simulink model "untitled2"  (R2018a)
settings: Solver=VariableStepAuto  StartTime=0.0  StopTime=10.0  RelTol=1e-3
undefined symbols (not defined in the file or in its folder): a, b, c, u0, x0
settings Model: Creator=adiravishankara  LastModifiedBy=adiravishankara

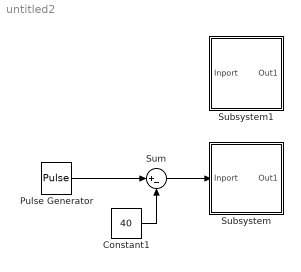
== system untitled2 ==
  Constant1 : Constant  Value=40
  Pulse Generator : DiscretePulseGenerator  PulseType=Time based  Period=10  PulseWidth=5
  Subsystem : Subsystem
  Subsystem1 : Subsystem
  Sum : Sum  Inputs=|+-
  wires:
  Pulse Generator/1 -> Sum/1
  Constant1/1 -> Sum/2
  Sum/1 -> Subsystem/1(Inport)

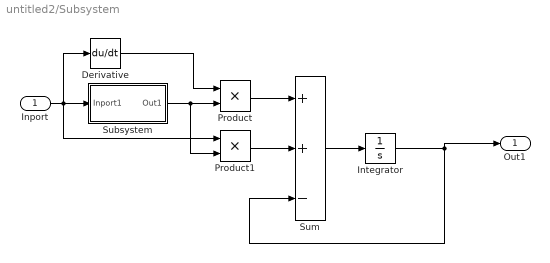
== system untitled2/Subsystem ==
  Inport : Inport
  Derivative : Derivative
  Integrator : Integrator
  Product : Product
  Product1 : Product
  Subsystem : Subsystem
  Sum : Sum  Inputs=++-
  Out1 : Outport
  wires:
  Product/1 -> Sum/1
  Sum/1 -> Integrator/1
  Subsystem/1(Out1) -> Product1/2, Product/2
  Integrator/1 -> Out1/1, Sum/3
  Inport/1 -> Product1/1, Derivative/1, Subsystem/1(Inport1)
  Product1/1 -> Sum/2
  Derivative/1 -> Product/1

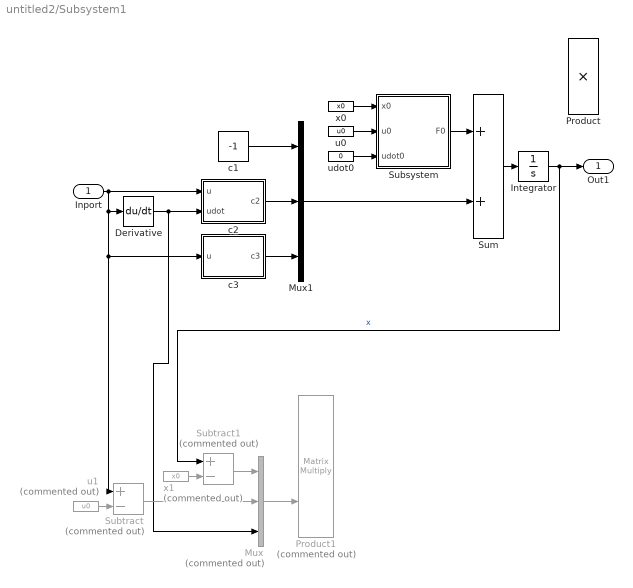
== system untitled2/Subsystem1 ==
  Inport : Inport
  Derivative : Derivative
  Integrator : Integrator
  Mux : Mux  Commented=on  Inputs=3
  Mux1 : Mux  Inputs=3
  Product : Product
  Product1 : Product  Commented=on  Multiplication=Matrix(*)
  Subsystem : Subsystem
  Subtract : Sum  Commented=on  Inputs=+-
  Subtract1 : Sum  Commented=on  Inputs=+-
  Sum : Sum
  c1 : Constant  Value=-1
  c2 : Subsystem
  c3 : Subsystem
  u0 : Constant  Value=u0
  u1 : Constant  Commented=on  Value=u0
  udot0 : Constant  Value=0
  x0 : Constant  Value=x0
  x1 : Constant  Commented=on  Value=x0
  Out1 : Outport
  wires:
  Integrator/1 -> Subtract1/1, Out1/1  "x"
  Sum/1 -> Integrator/1
  Mux/1 -> Product1/2
  Mux1/1 -> Sum/2
  c3/1(c3) -> Mux1/3
  c2/1(c2) -> Mux1/2
  c1/1 -> Mux1/1
  Subsystem/1(F0) -> Sum/1
  udot0/1 -> Subsystem/3(udot0)
  u0/1 -> Subsystem/2(u0)
  x0/1 -> Subsystem/1(x0)
  Inport/1 -> c2/1(u), Subtract/1, c3/1(u), Derivative/1
  Derivative/1 -> Mux/3, c2/2(udot)
  u1/1 -> Subtract/2
  Subtract/1 -> Mux/2
  Subtract1/1 -> Mux/1
  x1/1 -> Subtract1/2

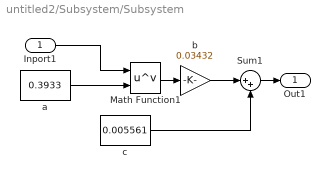
== system untitled2/Subsystem/Subsystem ==
  Inport1 : Inport
  Math Function1 : Math  Operator=pow  SaturateOnIntegerOverflow=on
  Sum1 : Sum  Inputs=|++
  a : Constant  Value=0.3933
  b : Gain  Gain=0.03432
  c : Constant  Value=0.005561
  Out1 : Outport
  wires:
  c/1 -> Sum1/2
  Sum1/1 -> Out1/1
  Math Function1/1 -> b/1
  Inport1/1 -> Math Function1/1
  b/1 -> Sum1/1
  a/1 -> Math Function1/2

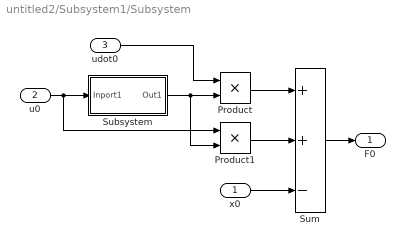
== system untitled2/Subsystem1/Subsystem ==
  x0 : Inport
  u0 : Inport  Port=2
  udot0 : Inport  Port=3
  Product : Product
  Product1 : Product
  Subsystem : Subsystem
  Sum : Sum  Inputs=++-
  F0 : Outport
  wires:
  Product/1 -> Sum/1
  Subsystem/1(Out1) -> Product1/2, Product/2
  u0/1 -> Product1/1, Subsystem/1(Inport1)
  Product1/1 -> Sum/2
  udot0/1 -> Product/1
  Sum/1 -> F0/1
  x0/1 -> Sum/3

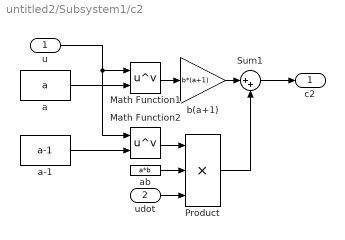
== system untitled2/Subsystem1/c2 ==
  u : Inport
  udot : Inport  Port=2
  Math Function1 : Math  Operator=pow  SaturateOnIntegerOverflow=on
  Math Function2 : Math  Operator=pow  SaturateOnIntegerOverflow=on
  Product : Product  Inputs=3
  Sum1 : Sum  Inputs=|++
  a : Constant  Value=a
  a-1 : Constant  Value=a-1
  ab : Constant  Value=a*b
  b(a+1) : Gain  Gain=b*(a+1)
  c2 : Outport
  wires:
  Sum1/1 -> c2/1
  Math Function1/1 -> b(a+1)/1
  u/1 -> Math Function2/1, Math Function1/1
  b(a+1)/1 -> Sum1/1
  a/1 -> Math Function1/2
  a-1/1 -> Math Function2/2
  Math Function2/1 -> Product/1
  ab/1 -> Product/2
  udot/1 -> Product/3
  Product/1 -> Sum1/2

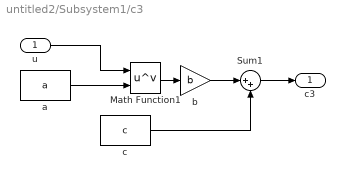
== system untitled2/Subsystem1/c3 ==
  u : Inport
  Math Function1 : Math  Operator=pow  SaturateOnIntegerOverflow=on
  Sum1 : Sum  Inputs=|++
  a : Constant  Value=a
  b : Gain  Gain=b
  c : Constant  Value=c
  c3 : Outport
  wires:
  a/1 -> Math Function1/2
  b/1 -> Sum1/1
  u/1 -> Math Function1/1
  Math Function1/1 -> b/1
  Sum1/1 -> c3/1
  c/1 -> Sum1/2

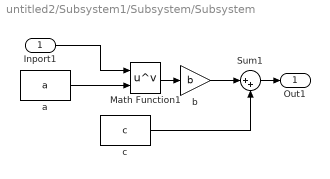
== system untitled2/Subsystem1/Subsystem/Subsystem ==
  Inport1 : Inport
  Math Function1 : Math  Operator=pow  SaturateOnIntegerOverflow=on
  Sum1 : Sum  Inputs=|++
  a : Constant  Value=a
  b : Gain  Gain=b
  c : Constant  Value=c
  Out1 : Outport
  wires:
  c/1 -> Sum1/2
  Sum1/1 -> Out1/1
  Math Function1/1 -> b/1
  Inport1/1 -> Math Function1/1
  b/1 -> Sum1/1
  a/1 -> Math Function1/2
